simulink model "GFM_referenceModel"  (R2023b)
settings: Solver=ode23  StartTime=0.0  StopTime=SimulationSetup.Solver.timeSimulationEnd  MaxStep=SimulationSetup.Solver.MaxStep  RelTol=SimulationSetup.Solver.RelTol
undefined symbols (not defined in the file): H, K_damping, Kdroop_V, Ki_CC, Kp_CC, Lconv1, Lg, Lv, Qref, Rconv1, Rg, Rv, Sbase, SimulationSetup, Vpeak, wf_PQ, wg
libraries: spsdq0toabcLib x1
settings Model: Creator=kauchr  LastModifiedBy=kauchr
settings DataIOCC: SaveFinalState=on  SaveOperatingPoint=on  SaveState=on

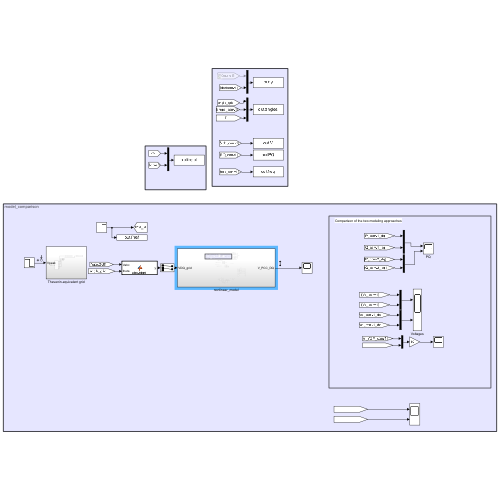
[thumbnail: Simulink's stored preview of the top-level diagram]
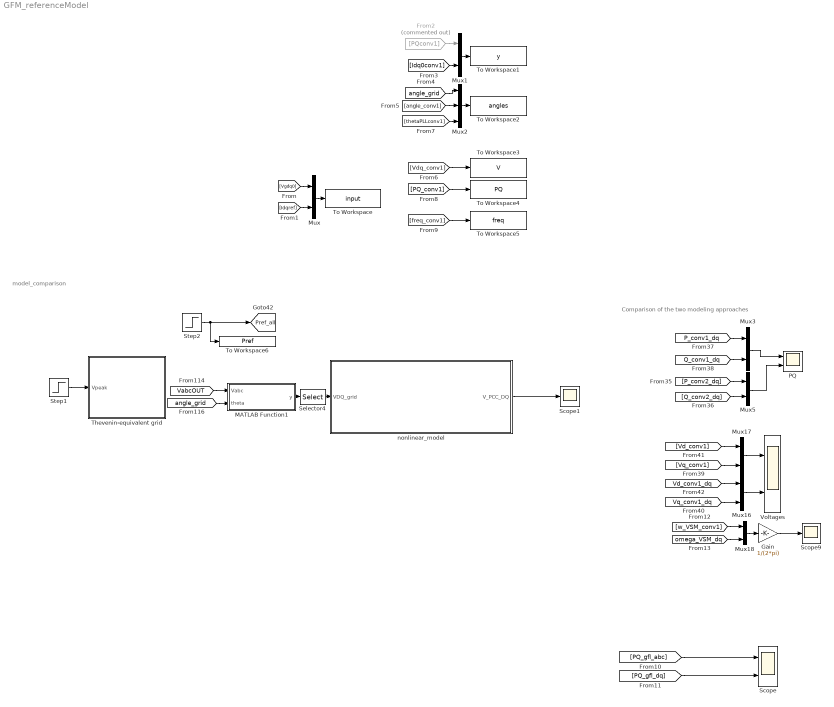
== system GFM_referenceModel ==
  note: model_comparison
  note: Comparison of the two modeling approaches
  From2 : From  Commented=on  GotoTag=PQconv1
  Gain : Gain  Gain=1/(2*pi)
  MATLAB Function1 : MATLAB Function  TreatAsAtomicUnit=on
  Mux{,1,3,5,16..18} (7 alike) : Mux  Inputs=2
  Mux2 : Mux  Inputs=3
  PQ : Scope  NumInputPorts=2
  Scope : Scope  NumInputPorts=2
  Scope1 : Scope
  Scope9 : Scope
  Selector4 : Selector  InputPortWidth=3  IndexOptions=Index vector (dialog)  Indices=[1 2]  OutputSizes=1
  Step1 : Step  Time=SimulationSetup.grid.voltageAmplitudeStep.Time  Before=SimulationSetup.grid.voltageAmplitudeStep.Values(1)  After=SimulationSetup.grid.voltageAmplitudeStep.Values(2)  SampleTime=0
  Step2 : Step  Time=SimulationSetup.converter1.Pref.Time  Before=SimulationSetup.converter1.Pref.Values(1)  After=SimulationSetup.converter1.Pref.Values(2)  SampleTime=0
  Thevenin-equivalent grid : Subsystem
  To Workspace : ToWorkspace  VariableName=input  SaveFormat=Timeseries  SampleTime=-1
  To Workspace1 : ToWorkspace  VariableName=y  SaveFormat=Timeseries  SampleTime=-1
  To Workspace2 : ToWorkspace  VariableName=angles  SaveFormat=Timeseries  SampleTime=-1
  To Workspace3 : ToWorkspace  VariableName=V  SaveFormat=Timeseries  SampleTime=-1
  To Workspace4 : ToWorkspace  VariableName=PQ  SaveFormat=Timeseries  SampleTime=-1
  To Workspace5 : ToWorkspace  VariableName=freq  SaveFormat=Timeseries  SampleTime=-1
  To Workspace6 : ToWorkspace  VariableName=Pref  SaveFormat=Timeseries  SampleTime=-1
  Voltages : Scope  NumInputPorts=2
  nonlinear_model : Subsystem
  tag scope: Pref_all=global
  wires:
  [Vgdq0] -> Mux/1
  [Idqref] -> Mux/2
  Mux/1 -> To Workspace/1
  Mux1/1 -> To Workspace1/1
  From2/1 -> Mux1/1
  [Idq0conv1] -> Mux1/2
  Mux2/1 -> To Workspace2/1
  [angle_grid] -> Mux2/1
  [angle_conv1] -> Mux2/2
  [Vdq_conv1] -> To Workspace3/1
  [thetaPLLconv1] -> Mux2/3
  [PQ_conv1] -> To Workspace4/1
  [freq_conv1] -> To Workspace5/1
  nonlinear_model/1(V_PCC_DQ) -> Scope1/1
  Selector4/1 -> nonlinear_model/1(VDQ_grid)
  [VabcOUT] -> MATLAB Function1/1(Vabc)
  [PQ_gfl_dq] -> Scope/2
  [PQ_gfl_abc] -> Scope/1
  Step2/1 -> To Workspace6/1, [Pref_all]
  [Vq_conv1] -> Mux17/2
  [Vd_conv1_dq] -> Mux16/1
  [Vq_conv1_dq] -> Mux16/2
  [Vd_conv1] -> Mux17/1
  [P_conv1_dq] -> Mux3/1
  [Q_conv1_dq] -> Mux3/2
  Mux5/1 -> PQ/2
  [Q_conv2_dq] -> Mux5/2
  [P_conv2_dq] -> Mux5/1
  Mux3/1 -> PQ/1
  Gain/1 -> Scope9/1
  Mux18/1 -> Gain/1
  [omega_VSM_dq] -> Mux18/2
  [w_VSM_conv1] -> Mux18/1
  Mux17/1 -> Voltages/1
  Mux16/1 -> Voltages/2
  Step1/1 -> Thevenin-equivalent grid/1(Vpeak)
  [angle_grid] -> MATLAB Function1/2(theta)
  MATLAB Function1/1(y) -> Selector4/1

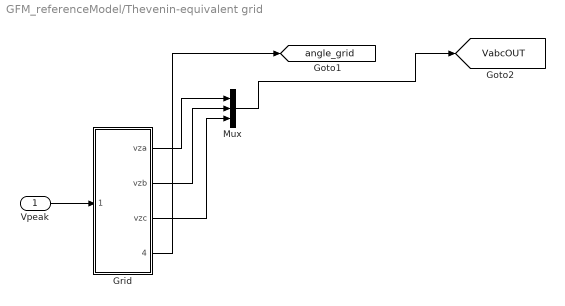
== system GFM_referenceModel/Thevenin-equivalent grid ==
  Vpeak : Inport
  Grid : Subsystem
  Mux : Mux  Inputs=3
  tag scope: VabcOUT=global, angle_grid=global
  wires:
  Grid/4(thetareal) -> [angle_grid]
  Grid/2(vzb) -> Mux/2
  Grid/3(vzc) -> Mux/3
  Mux/1 -> [VabcOUT]
  Grid/1(vza) -> Mux/1
  Vpeak/1 -> Grid/1(Vpeak)

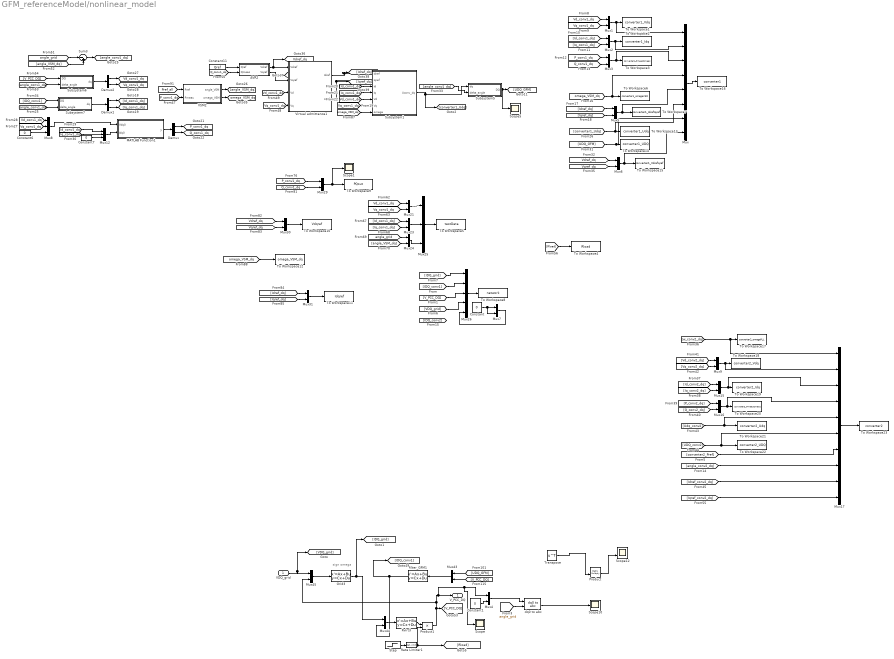
== system GFM_referenceModel/nonlinear_model ==
  note: sign omega
  VDQ_grid : Inport
  AVR2 : Subsystem
  Constant{,1,6..7} (4 alike) : Constant  Value=0
  Constant11 : Constant  Value=Qref
  Demux : Demux  Outputs=2
  Demux1 : Demux  Outputs=2
  Demux2 : Demux  Outputs=2
  Grid3 : StateSpace  A=[-Rg/Lg wg; -wg -Rg/Lg]  B=1/Lg*[eye(2),-eye(2)]  C=eye(2)  D=zeros(2,4)  InitialCondition=0  ContinuousStateAttributes='grid_IDQ'
  MATLAB Function1 : MATLAB Function  TreatAsAtomicUnit=on
  Mux : Mux  Inputs=[2 2 2 1 2 2 2 2]
  Mux{1..3,5..7,9,15..16,21,23..24,29..31} (15 alike) : Mux  Inputs=2
  Mux12 : Mux  Inputs=3
  Mux17 : Mux  Inputs=[1 2 2 2 2 2 1 1 1 1]
  Mux25 : Mux  Inputs=3
  Mux26 : Mux  Inputs=5
  Mux4 : Mux  Inputs=[2 1]
  Mux43 : Mux  Inputs=[2 2]
  Mux44 : Mux  Inputs=[2 2]
  Mux45 : Mux  Inputs=[2 2]
  Mux8 : Mux  Inputs=3
  Product : Product  Multiplication=Matrix(*)
  Product1 : Product
  Rate Limiter1 : RateLimiter  RisingSlewLimit=1000000  FallingSlewLimit=-1000000  SampleTimeMode=inherited
  Rvirt3 : StateSpace  A=[]  B=[]  C=[]  D=[eye(2),eye(2)]  InitialCondition=0  ContinuousStateAttributes='VDQ_PCC'
  Scope{,1,5,10} (4 alike) : Scope
  Scope12 : Scope  NumInputPorts=2
  Step : Step  Time=SimulationSetup.Load.Step.Time  Before=SimulationSetup.Load.Base  After=SimulationSetup.Load.Step.Value  SampleTime=0
  Subsystem1 : Subsystem
  Subsystem5 : Subsystem
  Subsystem6 : Subsystem
  Subsystem7 : Subsystem
  Sum3 : Sum  Inputs=|-+
  To Workspace1 : ToWorkspace  VariableName=converter1_Vdq  SaveFormat=Structure With Time  SampleTime=-1
  To Workspace10 : ToWorkspace  VariableName=Vdqref  SaveFormat=Timeseries  SampleTime=-1
      settings: Save2DSignal=2-D array (concatenate along first dimension)
  To Workspace11 : ToWorkspace  VariableName=Idqref  SaveFormat=Timeseries  SampleTime=-1
      settings: Save2DSignal=2-D array (concatenate along first dimension)
  To Workspace12 : ToWorkspace  VariableName=omega_VSM_dq  SaveFormat=Timeseries  SampleTime=-1
      settings: Save2DSignal=2-D array (concatenate along first dimension)
  To Workspace13 : ToWorkspace  VariableName=converter1_Udq  SaveFormat=Timeseries  SampleTime=-1
      settings: Save2DSignal=2-D array (concatenate along first dimension)
  To Workspace14 : ToWorkspace  VariableName=converter1_UDQ  SaveFormat=Timeseries  SampleTime=-1
      settings: Save2DSignal=2-D array (concatenate along first dimension)
  To Workspace15 : ToWorkspace  VariableName=converter1_Vdrefqref  SaveFormat=Timeseries  SampleTime=-1
      settings: Save2DSignal=2-D array (concatenate along first dimension)
  To Workspace16 : ToWorkspace  VariableName=converter1  SaveFormat=Structure With Time  SampleTime=-1
  To Workspace17 : ToWorkspace  VariableName=converter2_omegaPLL  SaveFormat=Timeseries  SampleTime=-1
      settings: Save2DSignal=2-D array (concatenate along first dimension)
  To Workspace18 : ToWorkspace  VariableName=converter2_Vdq  SaveFormat=Structure With Time  SampleTime=-1
  To Workspace19 : ToWorkspace  VariableName=converter2_Idq  SaveFormat=Structure With Time  SampleTime=-1
  To Workspace2 : ToWorkspace  VariableName=converter1_Idq  SaveFormat=Structure With Time  SampleTime=-1
  To Workspace20 : ToWorkspace  VariableName=converter2_PmeasQmeas  SaveFormat=Structure With Time  SampleTime=-1
  To Workspace21 : ToWorkspace  VariableName=converter2_Udq  SaveFormat=Timeseries  SampleTime=-1
      settings: Save2DSignal=2-D array (concatenate along first dimension)
  To Workspace22 : ToWorkspace  VariableName=converter2_UDQ  SaveFormat=Timeseries  SampleTime=-1
      settings: Save2DSignal=2-D array (concatenate along first dimension)
  To Workspace23 : ToWorkspace  VariableName=converter2  SaveFormat=Structure  SampleTime=-1
      settings: Save2DSignal=2-D array (concatenate along first dimension)
  To Workspace3 : ToWorkspace  VariableName=converter1_PmeasQmeas  SaveFormat=Structure With Time  SampleTime=-1
  To Workspace4 : ToWorkspace  VariableName=Rload  SaveFormat=Timeseries  SampleTime=-1
      settings: Save2DSignal=2-D array (concatenate along first dimension)
  To Workspace5 : ToWorkspace  VariableName=testData  SaveFormat=Structure With Time  SampleTime=-1
  To Workspace6 : ToWorkspace  VariableName=converter1_omegaVSM  SaveFormat=Timeseries  SampleTime=-1
      settings: Save2DSignal=2-D array (concatenate along first dimension)
  To Workspace7 : ToWorkspace  VariableName=converter1_IdrefIqref  SaveFormat=Timeseries  SampleTime=-1
      settings: Save2DSignal=2-D array (concatenate along first dimension)
  To Workspace8 : ToWorkspace  VariableName=network  SaveFormat=Timeseries  SampleTime=-1
      settings: Save2DSignal=2-D array (concatenate along first dimension)
  To Workspace9 : ToWorkspace  VariableName=PQout  SaveFormat=Timeseries  SampleTime=-1
      settings: Save2DSignal=2-D array (concatenate along first dimension)
  Transpose : Math  Operator=transpose
  VSM2 : Subsystem
  Virtual admittance1 : Subsystem
  dq0 to abc : spsdq0toabcLib/dq0 to abc  Alignment=90 degrees behind phase A axis
  filter_GFM1 : StateSpace  A=[-Rconv1/Lconv1 wg; -wg -Rconv1/Lconv1]  B=1/Lconv1*[eye(2),-eye(2)]  C=eye(2)  D=zeros(2,4)  InitialCondition=0  ContinuousStateAttributes='converter1_IDQ'
  V_PCC_DQ : Outport
  tag scope: P_conv1_dq=global, Q_conv1_dq=global, Vd_conv1_dq=global, Vdref_dq=global, Vq_conv1_dq=global, Vqref_dq=global, omega_VSM_dq=global
  wires:
  [Id_conv1_dq] -> Subsystem1/3(Id)
  Mux24/1 -> Mux25/3
  [Pref_all] -> VSM2/1(Pref)
  Mux29/1 -> Scope1/1, To Workspace9/1
  Mux12/1 -> MATLAB Function1/2(Idq0)
  Mux30/1 -> To Workspace10/1
  Demux/2 -> [Q_conv1_dq]
  Constant6/1 -> Mux8/3
  AVR2/1(Vdref) -> [Vdref_dq], Virtual admittance1/1(Vdref)
  [P_conv1_dq] -> VSM2/2(Pmeas)
  [Iq_conv1_dq] -> Mux23/2
  Demux/1 -> [P_conv1_dq]
  [Vq_conv1_dq] -> Subsystem1/6(Vq)
  [angle_VSM_dq] -> Mux24/2
  Mux31/1 -> To Workspace11/1
  Sum3/1 -> [angle_conv1_dq]
  [Q_conv1_dq] -> Mux29/2
  [Vd_conv1_dq] -> Mux8/1
  Mux8/1 -> MATLAB Function1/1(Vdq0)
  Constant7/1 -> Mux12/3
  Constant11/1 -> AVR2/1(Qref)
  Virtual admittance1/1(Idref) -> [Idref_dq], Subsystem1/1(Idref)
  [Vq_conv1_dq] -> Mux21/2
  AVR2/2(Vqref) -> [Vqref_dq], Virtual admittance1/2(Vqref)
  Demux1/1 -> [Id_conv1_dq]
  [Id_conv1_dq] -> Mux12/1
  [omega_VSM_dq] -> Subsystem1/7(omega)
  VSM2/1(angle_VSM) -> [angle_VSM_dq]
  [Vq_conv1_dq] -> Mux8/2
  Demux2/2 -> [Vq_conv1_dq]
  Demux1/2 -> [Iq_conv1_dq]
  [Iqref_dq] -> Mux31/2
  [Vd_conv1_dq] -> Subsystem1/5(Vd)
  [Vdref_dq] -> Mux30/1
  [omega_VSM_dq] -> To Workspace12/1
  [angle_VSM_dq] -> Sum3/2
  [Vd_conv1_dq] -> Virtual admittance1/3(Vd)
  [angle_grid] -> Sum3/1
  Demux2/1 -> [Vd_conv1_dq]
  [Q_conv1_dq] -> AVR2/2(Qmeas)
  [Vq_conv1_dq] -> Virtual admittance1/4(Vq)
  Mux23/1 -> Mux25/2
  [Iq_conv1_dq] -> Subsystem1/4(Iq)
  [angle_grid] -> Mux24/1
  [Id_conv1_dq] -> Mux23/1
  Mux21/1 -> Mux25/1
  [Vd_conv1_dq] -> Mux21/1
  [Iq_conv1_dq] -> Mux12/2
  VSM2/2(omega_VSM) -> [omega_VSM_dq]
  [Idref_dq] -> Mux31/1
  Mux25/1 -> To Workspace5/1
  [Vqref_dq] -> Mux30/2
  Virtual admittance1/2(Iqref) -> Subsystem1/2(Iqref), [Iqref_dq]
  [P_conv1_dq] -> Mux29/1
  Subsystem1/1(Uconv_dq) -> Subsystem5/1(dq), [converter1_Udq]
  Mux45/1 -> Grid3/1
  Mux43/1 -> filter_GFM1/1
  filter_GFM1/1 -> Mux44/2, [IDQ_conv1]
  Grid3/1 -> [IDQ_grid], Mux44/1
  Mux44/1 -> Rvirt3/1
  [UDQ_GFM] -> Mux43/1
  [V_PCC_DQ] -> Mux43/2
  Mux26/1 -> To Workspace8/1
  [V_PCC_DQ] -> Mux26/3
  [VDQ_grid] -> Mux26/4
  [IDQ_grid] -> Mux26/1
  Mux1/1 -> Mux/1, To Workspace1/1
  [Vq_conv1_dq] -> Mux1/2
  [Vd_conv1_dq] -> Mux1/1
  [Iq_conv1_dq] -> Mux2/2
  [Id_conv1_dq] -> Mux2/1
  Mux3/1 -> Mux/3, To Workspace3/1
  [Q_conv1_dq] -> Mux3/2
  [P_conv1_dq] -> Mux3/1
  [omega_VSM_dq] -> Mux/4, To Workspace6/1
  [Idref_dq] -> Mux5/1
  [Iqref_dq] -> Mux5/2
  Mux5/1 -> Mux/5, To Workspace7/1
  [converter1_Udq] -> Mux/6, To Workspace13/1
  [UDQ_GFM] -> Mux/7, To Workspace14/1
  Mux6/1 -> Mux/8, To Workspace15/1
  [Vqref_dq] -> Mux6/2
  [Vdref_dq] -> Mux6/1
  Mux2/1 -> Mux/2, To Workspace2/1
  Mux/1 -> To Workspace16/1
  [w_conv2_dq] -> Mux17/1, To Workspace17/1
  [Vd_conv2_dq] -> Mux9/1
  Mux9/1 -> Mux17/2, To Workspace18/1
  Mux15/1 -> Mux17/3, To Workspace19/1
  [P_conv2_dq] -> Mux16/1
  [Vq_conv2_dq] -> Mux9/2
  Mux16/1 -> Mux17/4, To Workspace20/1
  [Q_conv2_dq] -> Mux16/2
  [Iq_conv2_dq] -> Mux15/2
  [Id_conv2_dq] -> Mux15/1
  [Udq_conv2] -> Mux17/5, To Workspace21/1
  [UDQ_conv2] -> Mux17/6, To Workspace22/1
  Mux17/1 -> To Workspace23/1
  VDQ_grid/1 -> [VDQ_grid], Mux45/1
  [angle_conv1_dq] -> Subsystem5/2(delta_angle)
  Subsystem5/1(DQ) -> Scope5/1, [UDQ_GFM]
  [V_PCC_DQ] -> Subsystem6/1(DQ)
  [angle_conv1_dq] -> Subsystem6/2(delta_angle)
  Subsystem7/1(dq) -> Demux1/1
  [IDQ_conv1] -> Subsystem7/1(DQ)
  [angle_conv1_dq] -> Subsystem7/2(delta_angle)
  Subsystem6/1(dq) -> Demux2/1
  [angle_grid] -> dq0 to abc/2
  Mux4/1 -> dq0 to abc/1
  Constant1/1 -> Mux4/2
  dq0 to abc/1 -> Scope10/1
  [converter2_Pref] -> Mux17/7
  [angle_conv2_dq] -> Mux17/8
  Transpose/1 -> Product/2
  Product/1 -> Scope12/2
  Constant/1 -> Mux7/2, Mux7/1
  [Idref_conv2_dq] -> Mux17/9
  [Iqref_conv2_dq] -> Mux17/10
  [IDQ_conv1] -> Mux26/2
  [Rload] -> To Workspace4/1
  Step/1 -> Rate Limiter1/1
  Rvirt3/1 -> Product1/1
  Rate Limiter1/1 -> Product1/2, [Rload]
  Product1/1 -> [V_PCC_DQ], Mux45/2, Scope/1, Mux4/1, V_PCC_DQ/1
  Mux7/1 -> Mux26/5
  MATLAB Function1/1(y) -> Demux/1

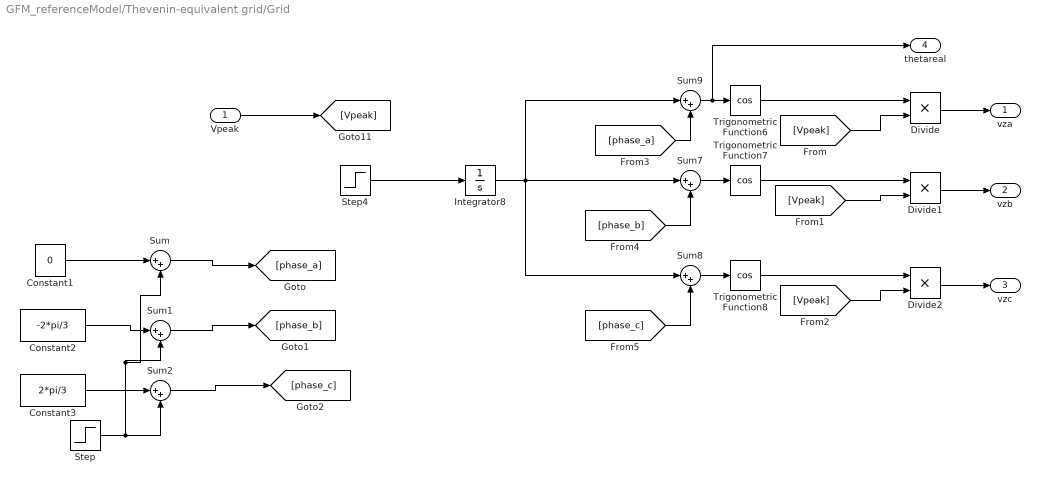
== system GFM_referenceModel/Thevenin-equivalent grid/Grid ==
  Vpeak : Inport
  Constant1 : Constant  Value=0
  Constant2 : Constant  Value=-2*pi/3
  Constant3 : Constant  Value=2*pi/3
  Divide : Product  Inputs=**
  Divide1 : Product  Inputs=**
  Divide2 : Product  Inputs=**
  Integrator8 : Integrator  ContinuousStateAttributes='grid_thetaGRID'
  Step : Step  Time=SimulationSetup.grid.PhaseStep.Time  Before=SimulationSetup.grid.PhaseStep.Values(1)  After=SimulationSetup.grid.PhaseStep.Values(2)  SampleTime=0
  Step4 : Step  Time=SimulationSetup.grid.FrequencyStep.Time  Before=SimulationSetup.grid.FrequencyStep.Values(1)  After=SimulationSetup.grid.FrequencyStep.Values(2)  SampleTime=0
  Sum{,1..2,7..9} (6 alike) : Sum  Inputs=|++
  Trigonometric Function6 : Trigonometry  Operator=cos
  Trigonometric Function7 : Trigonometry  Operator=cos
  Trigonometric Function8 : Trigonometry  Operator=cos
  vza : Outport
  vzb : Outport  Port=2
  vzc : Outport  Port=3
  thetareal : Outport  Port=4
  wires:
  Sum9/1 -> thetareal/1, Trigonometric Function6/1
  [phase_c] -> Sum8/2
  Integrator8/1 -> Sum8/1, Sum9/1, Sum7/1
  [phase_b] -> Sum7/2
  Sum7/1 -> Trigonometric Function7/1
  [phase_a] -> Sum9/2
  Sum8/1 -> Trigonometric Function8/1
  Trigonometric Function6/1 -> Divide/1
  Trigonometric Function7/1 -> Divide1/1
  Trigonometric Function8/1 -> Divide2/1
  Divide/1 -> vza/1
  Divide1/1 -> vzb/1
  Divide2/1 -> vzc/1
  [Vpeak] -> Divide/2
  [Vpeak] -> Divide1/2
  [Vpeak] -> Divide2/2
  Sum1/1 -> [phase_b]
  Sum/1 -> [phase_a]
  Constant1/1 -> Sum/1
  Constant2/1 -> Sum1/1
  Constant3/1 -> Sum2/1
  Sum2/1 -> [phase_c]
  Step/1 -> Sum/2, Sum1/2, Sum2/2
  Step4/1 -> Integrator8/1
  Vpeak/1 -> [Vpeak]

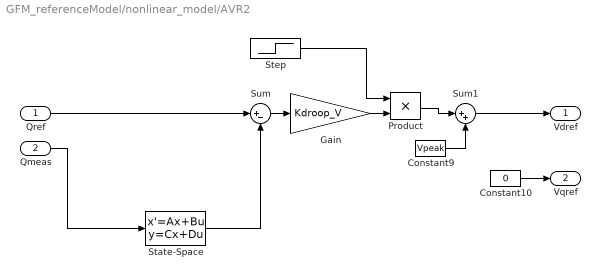
== system GFM_referenceModel/nonlinear_model/AVR2 ==
  Qref : Inport
  Qmeas : Inport  Port=2
  Constant10 : Constant  Value=0
  Constant9 : Constant  Value=Vpeak
  Gain : Gain  Gain=Kdroop_V
  Product : Product
  State-Space : StateSpace  A=-wf_PQ  B=wf_PQ  D=0  InitialCondition=0  ContinuousStateAttributes='converter1_xI_Vdroop'
  Step : Step  Time=SimulationSetup.converter1.VoltageCtrl.ActivationTime  SampleTime=0
  Sum : Sum  Inputs=|+-
  Sum1 : Sum  Inputs=|++
  Vdref : Outport
  Vqref : Outport  Port=2
  wires:
  Qref/1 -> Sum/1
  Constant9/1 -> Sum1/2
  Sum/1 -> Gain/1
  Qmeas/1 -> State-Space/1
  Sum1/1 -> Vdref/1
  Constant10/1 -> Vqref/1
  Product/1 -> Sum1/1
  Step/1 -> Product/1
  Gain/1 -> Product/2
  State-Space/1 -> Sum/2

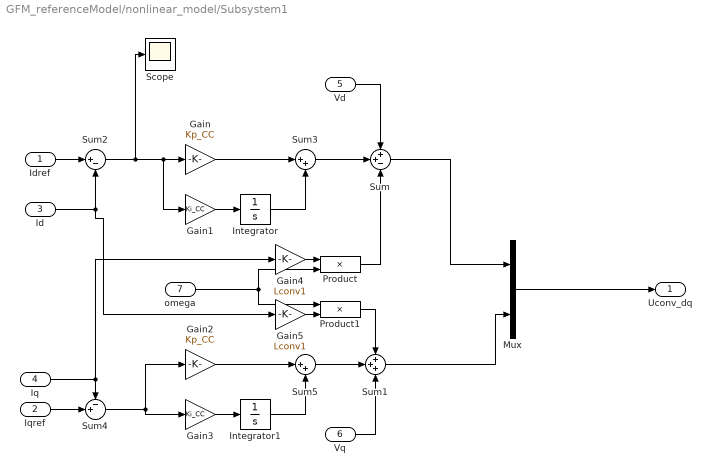
== system GFM_referenceModel/nonlinear_model/Subsystem1 ==
  Idref : Inport
  Iqref : Inport  Port=2
  Id : Inport  Port=3
  Iq : Inport  Port=4
  Vd : Inport  Port=5
  Vq : Inport  Port=6
  omega : Inport  Port=7
  Gain : Gain  Gain=Kp_CC
  Gain1 : Gain  Gain=Ki_CC
  Gain2 : Gain  Gain=Kp_CC
  Gain3 : Gain  Gain=Ki_CC
  Gain4 : Gain  Gain=Lconv1
  Gain5 : Gain  Gain=Lconv1
  Integrator : Integrator  ContinuousStateAttributes='converter1_xId_CC'
  Integrator1 : Integrator  ContinuousStateAttributes='converter1_xIq_CC'
  Mux : Mux  Inputs=2
  Product : Product
  Product1 : Product
  Scope : Scope
  Sum : Sum  Inputs=++-
  Sum1 : Sum  Inputs=+++
  Sum2 : Sum  Inputs=|+-
  Sum3 : Sum  Inputs=|++
  Sum4 : Sum  Inputs=-+|
  Sum5 : Sum  Inputs=|++
  Uconv_dq : Outport
  wires:
  Vd/1 -> Sum/1
  Vq/1 -> Sum1/3
  Sum/1 -> Mux/1
  Sum1/1 -> Mux/2
  Mux/1 -> Uconv_dq/1
  Idref/1 -> Sum2/1
  Id/1 -> Sum2/2, Gain5/1
  Sum2/1 -> Scope/1, Gain1/1, Gain/1
  Gain1/1 -> Integrator/1
  Integrator/1 -> Sum3/2
  Gain/1 -> Sum3/1
  Sum3/1 -> Sum/2
  Iqref/1 -> Sum4/2
  Iq/1 -> Gain4/1, Sum4/1
  Integrator1/1 -> Sum5/2
  Sum5/1 -> Sum1/2
  Gain3/1 -> Integrator1/1
  Gain2/1 -> Sum5/1
  Sum4/1 -> Gain2/1, Gain3/1
  Gain4/1 -> Product/1
  Product/1 -> Sum/3
  omega/1 -> Product/2, Product1/1
  Gain5/1 -> Product1/2
  Product1/1 -> Sum1/1

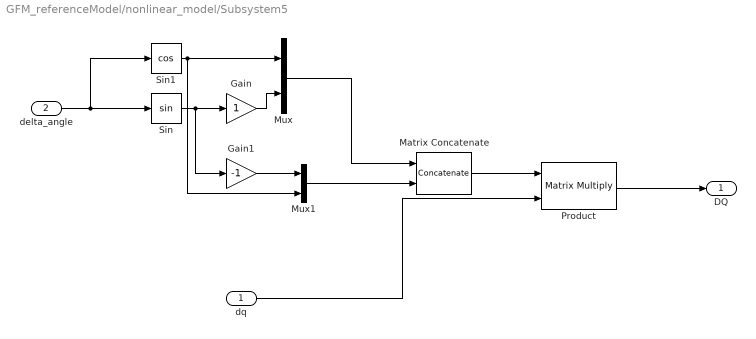
== system GFM_referenceModel/nonlinear_model/Subsystem5 ==
  dq : Inport
  delta_angle : Inport  Port=2
  Gain : Gain
  Gain1 : Gain  Gain=-1
  Matrix Concatenate : Concatenate  Mode=Multidimensional array  ConcatenateDimension=2
  Mux : Mux  Inputs=2
  Mux1 : Mux  Inputs=2
  Product : Product  Multiplication=Matrix(*)
  Sin : Trigonometry
  Sin1 : Trigonometry  Operator=cos
  DQ : Outport
  wires:
  Matrix Concatenate/1 -> Product/1
  dq/1 -> Product/2
  Product/1 -> DQ/1
  delta_angle/1 -> Sin1/1, Sin/1
  Sin1/1 -> Mux1/2, Mux/1
  Sin/1 -> Gain1/1, Gain/1
  Gain/1 -> Mux/2
  Mux/1 -> Matrix Concatenate/1
  Mux1/1 -> Matrix Concatenate/2
  Gain1/1 -> Mux1/1

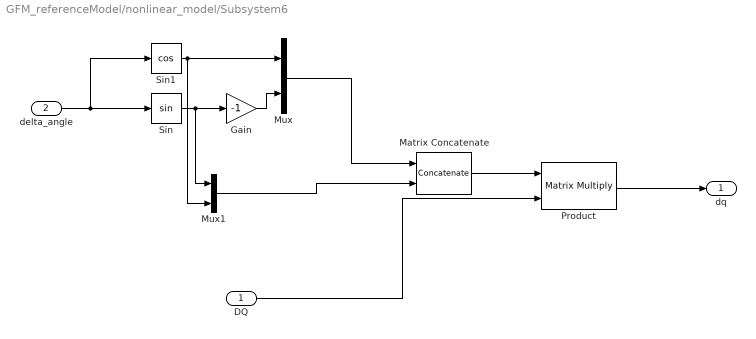
== system GFM_referenceModel/nonlinear_model/Subsystem6 ==
  DQ : Inport
  delta_angle : Inport  Port=2
  Gain : Gain  Gain=-1
  Matrix Concatenate : Concatenate  Mode=Multidimensional array  ConcatenateDimension=2
  Mux : Mux  Inputs=2
  Mux1 : Mux  Inputs=2
  Product : Product  Multiplication=Matrix(*)
  Sin : Trigonometry
  Sin1 : Trigonometry  Operator=cos
  dq : Outport
  wires:
  Matrix Concatenate/1 -> Product/1
  DQ/1 -> Product/2
  Product/1 -> dq/1
  delta_angle/1 -> Sin1/1, Sin/1
  Sin1/1 -> Mux1/2, Mux/1
  Sin/1 -> Mux1/1, Gain/1
  Gain/1 -> Mux/2
  Mux/1 -> Matrix Concatenate/1
  Mux1/1 -> Matrix Concatenate/2

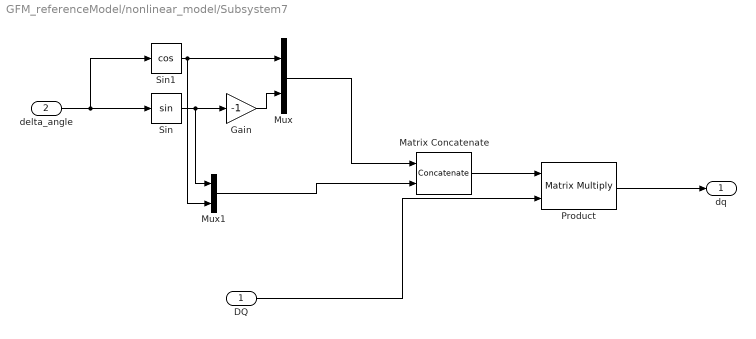
== system GFM_referenceModel/nonlinear_model/Subsystem7 ==
  DQ : Inport
  delta_angle : Inport  Port=2
  Gain : Gain  Gain=-1
  Matrix Concatenate : Concatenate  Mode=Multidimensional array  ConcatenateDimension=2
  Mux : Mux  Inputs=2
  Mux1 : Mux  Inputs=2
  Product : Product  Multiplication=Matrix(*)
  Sin : Trigonometry
  Sin1 : Trigonometry  Operator=cos
  dq : Outport
  wires:
  Matrix Concatenate/1 -> Product/1
  DQ/1 -> Product/2
  Product/1 -> dq/1
  delta_angle/1 -> Sin1/1, Sin/1
  Sin1/1 -> Mux1/2, Mux/1
  Sin/1 -> Mux1/1, Gain/1
  Gain/1 -> Mux/2
  Mux/1 -> Matrix Concatenate/1
  Mux1/1 -> Matrix Concatenate/2

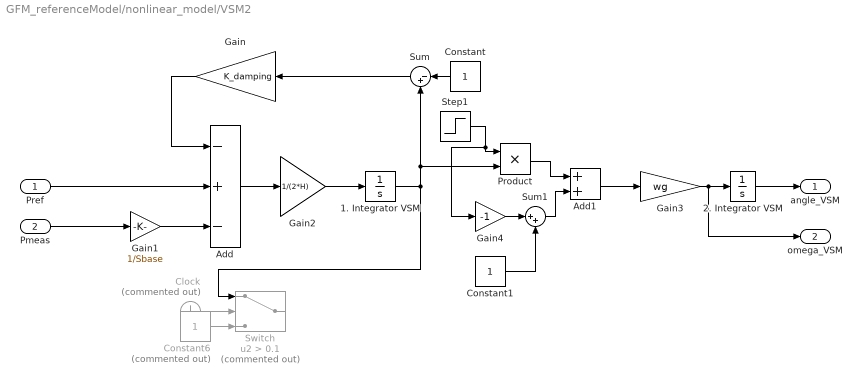
== system GFM_referenceModel/nonlinear_model/VSM2 ==
  Pref : Inport
  Pmeas : Inport  Port=2
  1. Integrator VSM : Integrator  ContinuousStateAttributes='converter1_xI_vsm'
  2. Integrator VSM : Integrator  ContinuousStateAttributes='converter1_thetaVSM'
  Add : Sum  Inputs=-+-
  Add1 : Sum
  Clock : Clock  Commented=on
  Constant : Constant
  Constant1 : Constant
  Constant6 : Constant  Commented=on
  Gain : Gain  Gain=K_damping
  Gain1 : Gain  Gain=1/Sbase
  Gain2 : Gain  Gain=1/(2*H)
  Gain3 : Gain  Gain=wg
  Gain4 : Gain  Gain=-1
  Product : Product
  Step1 : Step  Time=SimulationSetup.converter1.FreqCtrl.ActivationTime  SampleTime=0
  Sum : Sum  Inputs=|-+
  Sum1 : Sum  Inputs=|++
  Switch : Switch  Commented=on  Criteria=u2 > Threshold  Threshold=0.1  SaturateOnIntegerOverflow=off  InputSameDT=off
  angle_VSM : Outport
  omega_VSM : Outport  Port=2
  wires:
  Pmeas/1 -> Gain1/1
  Gain2/1 -> 1. Integrator VSM/1
  Pref/1 -> Add/2
  Gain1/1 -> Add/3
  Add/1 -> Gain2/1
  1. Integrator VSM/1 -> Product/2, Sum/2, Switch/1
  Constant/1 -> Sum/1
  Sum/1 -> Gain/1
  Gain/1 -> Add/1
  Gain3/1 -> omega_VSM/1, 2. Integrator VSM/1
  2. Integrator VSM/1 -> angle_VSM/1
  Clock/1 -> Switch/2
  Constant6/1 -> Switch/3
  Add1/1 -> Gain3/1
  Product/1 -> Add1/1
  Step1/1 -> Gain4/1, Product/1
  Gain4/1 -> Sum1/1
  Sum1/1 -> Add1/2
  Constant1/1 -> Sum1/2

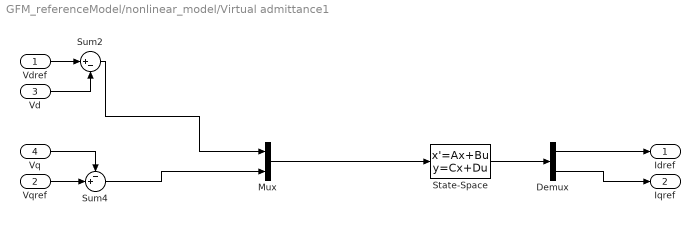
== system GFM_referenceModel/nonlinear_model/Virtual admittance1 ==
  Vdref : Inport
  Vqref : Inport  Port=2
  Vd : Inport  Port=3
  Vq : Inport  Port=4
  Demux : Demux  Outputs=2
  Mux : Mux  Inputs=2
  State-Space : StateSpace  A=[-Rv/Lv, wg; -wg, -Rv/Lv]  B=[1 0; 0 1]  C=1/Lv*eye(2)  D=zeros(2,2)  InitialCondition=0  ContinuousStateAttributes={'converter1_xId_VA','converter1_xIq_VA'}
  Sum2 : Sum  Inputs=|+-
  Sum4 : Sum  Inputs=-+|
  Idref : Outport
  Iqref : Outport  Port=2
  wires:
  Vdref/1 -> Sum2/1
  Vd/1 -> Sum2/2
  Vqref/1 -> Sum4/2
  Vq/1 -> Sum4/1
  Sum2/1 -> Mux/1
  Sum4/1 -> Mux/2
  Mux/1 -> State-Space/1
  State-Space/1 -> Demux/1
  Demux/1 -> Idref/1
  Demux/2 -> Iqref/1

== matlab function GFM_referenceModel/nonlinear_model/MATLAB Function1 ==
  data: Vdq0 input; y output; Idq0 input
function y = PQcalculation(Vdq0,Idq0)
 % alignment with d-axis
y =3/2*([Vdq0(1)*Idq0(1)+Vdq0(2)*Idq0(2)+2*Vdq0(3)*Idq0(3);Vdq0(2)*Idq0(1)-Vdq0(1)*Idq0(2);]);

== matlab function GFM_referenceModel/MATLAB Function1 ==
  data: Vabc input; y output; theta input
function y = abc2dq0(Vabc,theta)
 % alignment with d-axis
y =2/3*([cos(theta), cos(theta-2*pi/3),cos(theta+2*pi/3); -sin(theta), -sin(theta-2*pi/3), -sin(theta+2*pi/3); sqrt(0.5),sqrt(0.5),sqrt(0.5) ])*[Vabc(1);Vabc(2);Vabc(3)];
